simulink model "funcionesdetranferencia"  (R2015a)
settings: Solver=ode45  StartTime=0.0  StopTime=10.0  RelTol=1e-3
settings Model: Creator=jeanb  LastModifiedBy=jeanb

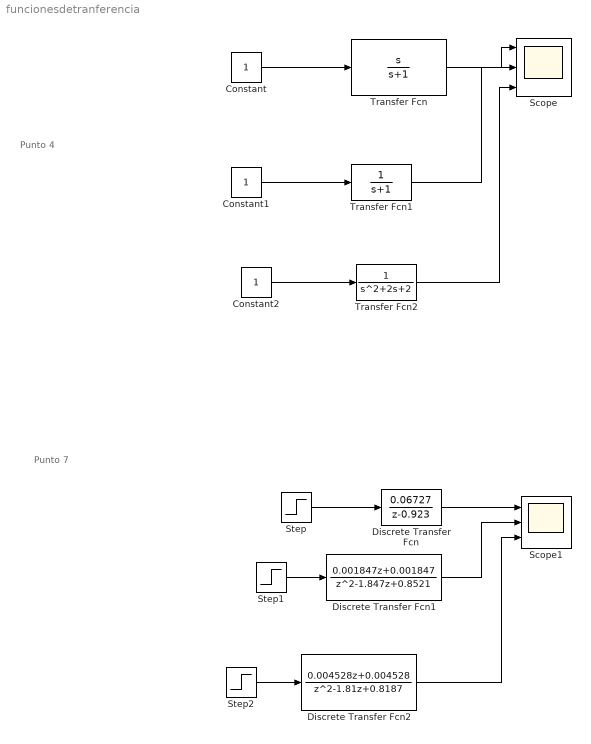
== system funcionesdetranferencia ==
  note: Punto 7
  note: Punto 4
  Constant : Constant
  Constant1 : Constant
  Constant2 : Constant
  Discrete Transfer Fcn : DiscreteTransferFcn  Numerator=[0.06727]  Denominator=[1 -0.923]  SampleTime=0.1
  Discrete Transfer Fcn1 : DiscreteTransferFcn  Numerator=[0.001847 0.001847]  Denominator=[1 -1.847 0.8521]  SampleTime=0.1
  Discrete Transfer Fcn2 : DiscreteTransferFcn  Numerator=[0.004528 0.004528]  Denominator=[1 -1.81 0.8187]  SampleTime=0.1
  Scope : Scope  NumInputPorts=3
      settings: YMin=-5~-5~-5  YMax=5~5~5
  Scope1 : Scope  NumInputPorts=3
      settings: TimeRange=10  YMin=-5~-5~-5  YMax=5~5~5
  Step : Step  Time=0  SampleTime=0
  Step1 : Step  Time=0  SampleTime=0
  Step2 : Step  Time=0  SampleTime=0
  Transfer Fcn : TransferFcn  Numerator=[1 0]  Denominator=[1 1]
  Transfer Fcn1 : TransferFcn  Denominator=[1 1 ]
  Transfer Fcn2 : TransferFcn  Denominator=[1 2 2 ]
  wires:
  Transfer Fcn/1 -> Scope/1
  Constant/1 -> Transfer Fcn/1
  Constant1/1 -> Transfer Fcn1/1
  Transfer Fcn1/1 -> Scope/2
  Constant2/1 -> Transfer Fcn2/1
  Transfer Fcn2/1 -> Scope/3
  Discrete Transfer Fcn/1 -> Scope1/1
  Step/1 -> Discrete Transfer Fcn/1
  Step1/1 -> Discrete Transfer Fcn1/1
  Discrete Transfer Fcn1/1 -> Scope1/2
  Step2/1 -> Discrete Transfer Fcn2/1
  Discrete Transfer Fcn2/1 -> Scope1/3
